simulink model "ADAS_Simulink_Model"  (R2026a)
settings: Solver=VariableStepAuto
libraries: simulink x1
settings Model: Creator=mushu  LastModifiedBy=mushu

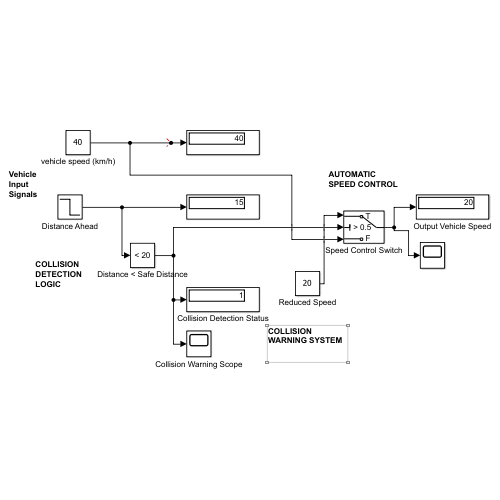
[thumbnail: Simulink's stored preview of the top-level diagram]
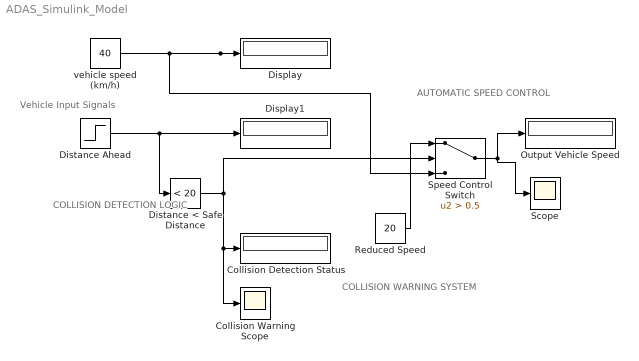
== system ADAS_Simulink_Model ==
  note: COLLISION WARNING SYSTEM
  note: AUTOMATIC SPEED CONTROL
  note: COLLISION DETECTION LOGIC
  note: Vehicle Input Signals
  Collision Detection Status : Display
  Collision Warning Scope : Scope
      settings: ActiveDisplayYMinimum=-0.12499999999999997  ActiveDisplayYMaximum=1.125
  Display : Display
  Display1 : Display
  Distance < Safe Distance : simulink/Logic and Bit Operations/Compare To Constant  relop=<  const=20  OutDataTypeStr=boolean
  Distance Ahead : Step  Time=5  InitialValue=25  FinalValue=15  SampleTime=0
  Output Vehicle Speed : Display
  Reduced Speed : Constant  Value=20
  Scope : Scope
      settings: ActiveDisplayYMinimum=17.5  ActiveDisplayYMaximum=42.5
  Speed Control Switch : Switch  Criteria=u2 > Threshold  Threshold=0.5  SaturateOnIntegerOverflow=off  InputSameDT=off
  vehicle speed (km/h) : Constant  Value=40
  wires:
  vehicle speed (km/h)/1 -> Speed Control Switch/3, Display/1
  Distance Ahead/1 -> Distance < Safe Distance/1, Display1/1
  Distance < Safe Distance/1 -> Speed Control Switch/2, Collision Warning Scope/1, Collision Detection Status/1
  Reduced Speed/1 -> Speed Control Switch/1
  Speed Control Switch/1 -> Output Vehicle Speed/1, Scope/1
